simulink model "UAVmodel"  (R2020a)
settings: Solver=FixedStepDiscrete  StartTime=0.0  StopTime=50  FixedStep=0.1  RelTol=1e-3  EnableMultiTasking=on
settings Model: Creator=anthonyabibadra  LastModifiedBy=anthonyabibadra
settings SolverCC: AutoInsertRateTranBlk=on
settings DataIOCC: LimitDataPoints=on
settings OptimizationCC: LifeSpan=inf
settings DebuggingCC: AllowSymbolicDim=off  SFUnexpectedBacktrackingDiag=warning  SFNoUnconditionalDefaultTransitionDiag=warning  SFExecutionAtInitializationDiag=none  ArithmeticOperatorsInVariantConditions=warning
settings SFSimCC: SimUseLocalCustomCode=off  CustomCodeUndefinedFunction=UseInterfaceOnly
settings RTWCC: RTWUseLocalCustomCode=off
settings CodeAppCC: StateflowObjectComments=on
settings GRTTargetCC: TargetLangStandard=C89/C90 (ANSI)
settings ConfigComp: CovMetricSettings=dw  CovHtmlReporting=on  CovSaveCumulativeToWorkspaceVar=on  CovSaveSingleToWorkspaceVar=on  CovShowResultsExplorer=off  CovExternalEMLEnable=off  CovSFcnEnable=off

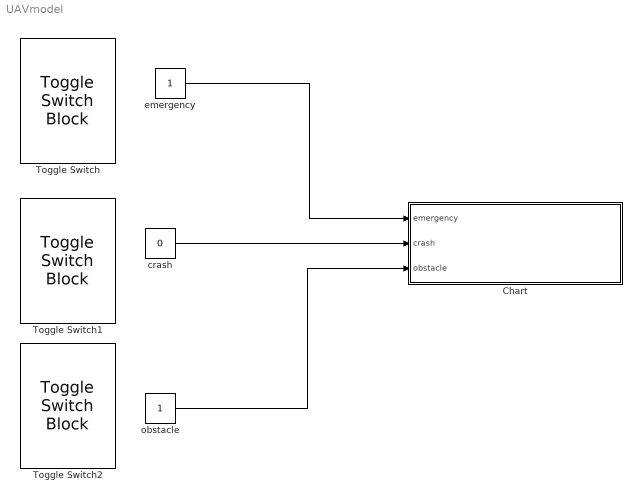
== system UAVmodel ==
  Chart : Stateflow chart  TreatAsAtomicUnit=on
  Toggle Switch : ToggleSwitchBlock
      settings: Values={{'Off', 'On'}, [0 1]}
  Toggle Switch1 : ToggleSwitchBlock
      settings: Values={{'Off', 'On'}, [0 1]}
  Toggle Switch2 : ToggleSwitchBlock
      settings: Values={{'Off', 'On'}, [0 1]}
  crash : Constant  Value=0
  emergency : Constant
  obstacle : Constant
  wires:
  emergency/1 -> Chart/1(emergency)
  crash/1 -> Chart/2(crash)
  obstacle/1 -> Chart/3(obstacle)

== stateflow chart UAVmodel/Chart ==
  state DroneReady
    entry:
    battery = 100
    latitude = 1
    longitude = 2
  state CheckLocation
  state TakeOff
    entry:
    altitude =0
    during:
    altitude = altitude +10
    battery = battery - 0.1
  state ObtscaleAvoidance
  state ReachDesiredAltitude
    entry:
    altitude = 150
    during:
    battery = battery -0.1
  state IncreaseAltitude
    during:
    altitude = altitude -0.1
    battery = battery -0.1
  state StopEngine
    during:
    altitude = altitude - 50
  state EmergencyMode
  state HorizontalFlight
    during:
    battery = battery -0.1
    latitude = latitude + 1
    longitude = longitude + 1
  state DecreaseAltitude
    during:
    altitude = altitude -0.1
    battery = battery -0.1
  state DroneCrashed
  state LowerAltitude
    on after(1 ,sec):
    altitude = altitude - 5 ;
    during:
    battery = battery -0.1
  state Inspect
    state Fly
      during:
      latitude = latitude + 1
      longitude = longitude + 1
      battery = battery -0.1
    state TakePicture
      image = image + 1
      during:
      battery = battery -0.1
    TakePicture -> Fly : [image> 0]{latitude = latitude + 1}
    Fly -> TakePicture [order 2] : [latitude == 5 & longitude == 6]
  state IncreaseAlt
    during:
    battery = battery -0.1
    altitude = altitude +5
  state FlyToBase
    during:
    battery = battery -0.1
    latitude = latitude -1
    longitude = longitude -1
  state DecreaseAlt
    during:
    battery = battery -0.1
    altitude = altitude - 5
  state StartLanding
    during:
    battery = battery -0.1
    altitude = altitude - 1
  state DroneLanded
  TakeOff -> ObtscaleAvoidance [order 3] : [obstacle == 1]
  ObtscaleAvoidance -> TakeOff [order 1] : [obstacle == 0]
  (default) -> DroneReady
  DroneReady -> CheckLocation : [battery > 80]
  CheckLocation -> TakeOff : [latitude ==1 & longitude == 2]
  TakeOff -> EmergencyMode [order 2] : [emergency == 1]
  TakeOff -> ReachDesiredAltitude [order 1] : [altitude == 150]
  ReachDesiredAltitude -> EmergencyMode [order 2] : [emergency == 1]
  ReachDesiredAltitude -> ObtscaleAvoidance [order 3] : [obstacle ==1]
  ObtscaleAvoidance -> ReachDesiredAltitude [order 2] : [obstacle == 0]
  ReachDesiredAltitude -> HorizontalFlight [order 1] : [after(2,sec)]
  IncreaseAltitude -> HorizontalFlight [order 1] : [altitude ==150]
  IncreaseAltitude -> ObtscaleAvoidance [order 3] : [obstacle == 1]
  HorizontalFlight -> IncreaseAltitude [order 1] : [altitude < 150 ]
  ObtscaleAvoidance -> IncreaseAltitude [order 3] : [obstacle == 0]
  IncreaseAltitude -> EmergencyMode [order 2] : [emergency ==1]
  EmergencyMode -> StopEngine [order 1] : [crash == 1]
  HorizontalFlight -> EmergencyMode [order 5] : [emergency ==1 ]
  EmergencyMode -> FlyToBase [order 2] : [crash == 0]{latitude =1; longitude=2; altitude = 50 }
  IncreaseAlt -> EmergencyMode [order 2] : [emergency == 1]
  Fly -> EmergencyMode [order 1] : [emergency == 1]
  LowerAltitude -> EmergencyMode [order 3] : [emergency ==1]
  DecreaseAltitude -> EmergencyMode [order 2] : [emergency ==1]
  StopEngine -> DroneCrashed : [altitude == 0]
  FlyToBase -> StopEngine [order 2] : [crash == 1]
  HorizontalFlight -> ObtscaleAvoidance [order 6] : [obstacle == 1]
  HorizontalFlight -> ObtscaleAvoidance [order 2] : [obstacle == 1]
  ObtscaleAvoidance -> HorizontalFlight [order 5] : [obstacle == 0]
  HorizontalFlight -> LowerAltitude [order 4] : [latitude==3 & longitude ==4]
  HorizontalFlight -> DecreaseAltitude [order 3] : [altitude > 150]
  DecreaseAltitude -> HorizontalFlight [order 1] : [altitude == 150]
  DecreaseAltitude -> ObtscaleAvoidance [order 3] : [obstacle == 1]
  ObtscaleAvoidance -> DecreaseAltitude [order 4] : [obstacle == 0]
  LowerAltitude -> ObtscaleAvoidance [order 2] : [obstacle == 1]
  ObtscaleAvoidance -> LowerAltitude [order 6] : [obstacle == 0]
  LowerAltitude -> Fly [order 1] : [altitude == 100]
  Fly -> ObtscaleAvoidance [order 4] : [obstacle == 1]
  ObtscaleAvoidance -> Fly [order 7] : [obstacle == 0]
  Fly -> IncreaseAlt [order 3] : [latitude == 25 & longitude == 25]
  IncreaseAlt -> ObtscaleAvoidance [order 3] : [obstacle == 1]
  ObtscaleAvoidance -> IncreaseAlt [order 8] : [obstacle == 0]
  IncreaseAlt -> FlyToBase [order 1] : [altitude == 150]{latitude = latitude -1}
  FlyToBase -> ObtscaleAvoidance [order 3] : [obstacle == 1]
  ObtscaleAvoidance -> FlyToBase [order 9] : [obstacle == 0]
  FlyToBase -> DecreaseAlt [order 1] : [latitude == 1 & longitude ==2]
  DecreaseAlt -> ObtscaleAvoidance [order 2] : [obstacle == 1]
  ObtscaleAvoidance -> DecreaseAlt [order 10] : [obstacle == 0]
  DecreaseAlt -> StartLanding [order 1] : [altitude == 20]
  StartLanding -> ObtscaleAvoidance [order 2] : [obstacle == 1]
  ObtscaleAvoidance -> StartLanding [order 11] : [obstacle == 0]
  StartLanding -> DroneLanded [order 1] : [altitude == 0]
  data: battery local double =100; altitude local =0; latitude local; longitude local; image local =0; emergency input; crash input; obstacle input
